simulink library "LM_LIB"  (R2019b)
settings: Solver=VariableStepAuto  StartTime=0.0  StopTime=10.0  RelTol=1e-3
undefined symbols (not defined in the file): P_LM_FusBLParFiltP, P_LM_FusParC0Index, P_LM_FusParC1Index, P_LM_FusParC2Index, P_LM_FusParC3Index, P_LM_OTLBufTPMinPntNum, P_LM_OTLBufTPSPosMinDis, P_LM_OTLRearMaxDis, P_LM_OTLTPNum
libraries: simulink x84, $bdroot x3
(part 1 of 5)
settings Model: Creator=GW00166374  LastModifiedBy=GW00166374

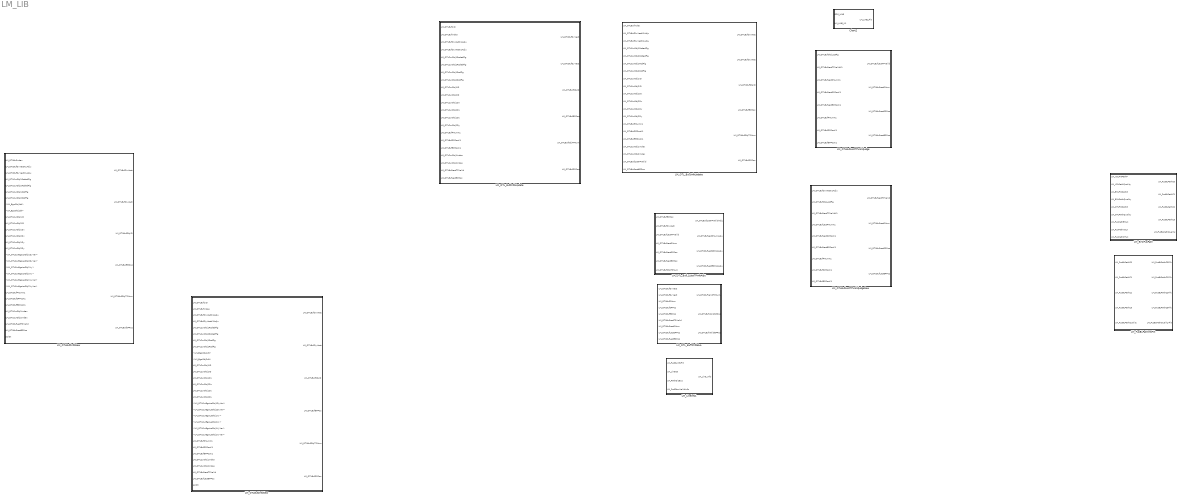
== system LM_LIB ==
  Chart2 : Stateflow chart  TreatAsAtomicUnit=on
  LM_EVOFusPath : Subsystem
  LM_FusBLPathInfoFilt : Subsystem
  LM_LineInfo1 : Subsystem
  LM_OTLBuf1InfoNew : Subsystem
  LM_OTLBuf2InfoNew : Subsystem
  LM_OTLBufLostTPValidJudge : Subsystem
  LM_OTLBufLostTPValidJudgeNew : Subsystem
  LM_OTL_Buf1InfoUpdate : Subsystem
  LM_OTL_Buf2InfoUpdate : Subsystem
  LM_OTL_BufL1LastTPInfoAdju : Subsystem
  LM_OTL_BufTPInfoEva : Subsystem

== system LM_LIB/LM_EVOFusPath ==
  LM_VSLFntPathP : Inport
  LM_VSLPathQuality : Inport  Port=2
  LM_EMLFntPathP : Inport  Port=3
  LM_EMLPathQuality : Inport  Port=4
  LM_OTLFntPathP : Inport  Port=5
  LM_OTLPathQuality : Inport  Port=6
  LM_FusPathEMLK : Inport  Port=7
  LM_FusPathVSLK : Inport  Port=8
  LM_FusPathOTLK : Inport  Port=9
  LM_FusBLPathC0Calc : Subsystem
  LM_FusBLPathC1Calc : Subsystem
  LM_FusBLPathC2Calc : Subsystem
  LM_FusBLPathC3Calc : Subsystem
  LM_FusBLPathQualityCalc : Stateflow chart  BlockKeywords=__PRM__SERIALIZED__DATA__:Stateflow Chart,Stateflow Diagram  TreatAsAtomicUnit=on
  LM_FusBLPathC0 : Outport
  LM_FusBLPathC1 : Outport  Port=2
  LM_FusBLPathC2 : Outport  Port=3
  LM_FusBLPathC3 : Outport  Port=4
  LM_FusBLPathQuality : Outport  Port=5
  wires:
  LM_FusBLPathQualityCalc/1(LM_FusBLPathQuality) -> LM_FusBLPathQuality/1, [LM_FusBLPathQuality]
  LM_FusBLPathC3Calc/1(LM_FusBLPathC3) -> LM_FusBLPathC3/1
  LM_FusBLPathC2Calc/1(LM_FusBLPathC2) -> LM_FusBLPathC2/1
  LM_FusBLPathC1Calc/1(LM_FusBLPathC1) -> LM_FusBLPathC1/1
  LM_FusBLPathC0Calc/1(LM_FusBLPathC0) -> LM_FusBLPathC0/1
  LM_OTLPathQuality/1 -> LM_FusBLPathQualityCalc/3(LM_OTLPathQuality)
  LM_EMLPathQuality/1 -> LM_FusBLPathQualityCalc/1(LM_EMLPathQuality)
  LM_VSLPathQuality/1 -> LM_FusBLPathQualityCalc/2(LM_VSLPathQuality)
  LM_FusPathOTLK/1 -> LM_FusBLPathC3Calc/7(LM_FusPathOTLK), LM_FusBLPathC2Calc/7(LM_FusPathOTLK), LM_FusBLPathC1Calc/7(LM_FusPathOTLK), LM_FusBLPathC0Calc/7(LM_FusPathOTLK), LM_FusBLPathQualityCalc/6(LM_FusPathOTLK)
  LM_FusPathVSLK/1 -> LM_FusBLPathC3Calc/6(LM_FusPathVSLK), LM_FusBLPathC2Calc/6(LM_FusPathVSLK), LM_FusBLPathC1Calc/6(LM_FusPathVSLK), LM_FusBLPathC0Calc/6(LM_FusPathVSLK), LM_FusBLPathQualityCalc/5(LM_FusPathVSLK)
  LM_FusPathEMLK/1 -> LM_FusBLPathC3Calc/5(LM_FusPathEMLK), LM_FusBLPathC2Calc/5(LM_FusPathEMLK), LM_FusBLPathC1Calc/5(LM_FusPathEMLK), LM_FusBLPathC0Calc/5(LM_FusPathEMLK), LM_FusBLPathQualityCalc/4(LM_FusPathEMLK)
  LM_OTLFntPathP/1 -> LM_FusBLPathC1Calc/4(LM_OTLPathP), LM_FusBLPathC2Calc/4(LM_OTLPathP), LM_FusBLPathC3Calc/4(LM_OTLPathP), LM_FusBLPathC0Calc/4(LM_OTLPathP)
  LM_EMLFntPathP/1 -> LM_FusBLPathC1Calc/3(LM_EMLPathP), LM_FusBLPathC2Calc/3(LM_EMLPathP), LM_FusBLPathC3Calc/3(LM_EMLPathP), LM_FusBLPathC0Calc/3(LM_EMLPathP)
  LM_VSLFntPathP/1 -> LM_FusBLPathC0Calc/2(LM_VSLPathP), LM_FusBLPathC1Calc/2(LM_VSLPathP), LM_FusBLPathC2Calc/2(LM_VSLPathP), LM_FusBLPathC3Calc/2(LM_VSLPathP)
  [LM_FusBLPathQuality] -> LM_FusBLPathC0Calc/1(LM_FusBLPathQuality), LM_FusBLPathC1Calc/1(LM_FusBLPathQuality), LM_FusBLPathC2Calc/1(LM_FusBLPathQuality), LM_FusBLPathC3Calc/1(LM_FusBLPathQuality)

== system LM_LIB/LM_FusBLPathInfoFilt ==
  LM_FusBLPathC0 : Inport
  LM_FusBLPathC1 : Inport  Port=2
  LM_FusBLPathC2 : Inport  Port=3
  LM_FusBLPathC3 : Inport  Port=4
  LM_FusBLPathQuality : Inport  Port=5
  LM_FusBLPathQuliatyFilt : Subsystem
  LM_Fus_BLFntPathC0Filt : Subsystem
  LM_Fus_BLPath3C3Filt : Subsystem
  LM_Fus_BLPathC1Filt : Subsystem
  LM_Fus_BLPathC2Filt : Subsystem
  Unit Delay{,1..4} (5 alike) : UnitDelay  SampleTime=-1  HasFrameUpgradeWarning=on
  LM_FusBLPathC0Filt : Outport
  LM_FusBLPathC1Filt : Outport  Port=2
  LM_FusBLPathC2Filt : Outport  Port=3
  LM_FusBLPathC3Filt : Outport  Port=4
  LM_FusBLPathQualityFilt : Outport  Port=5
  wires:
  LM_FusBLPathQuliatyFilt/1(LM_FusBLPathQualityFilt) -> Unit Delay4/1, LM_FusBLPathQualityFilt/1
  LM_Fus_BLPath3C3Filt/1(LM_FusBLPathC3Filt) -> Unit Delay3/1, LM_FusBLPathC3Filt/1
  Unit Delay3/1 -> LM_Fus_BLPath3C3Filt/4(LM_FusBLPathC3K1)
  LM_FusBLPathC3/1 -> LM_Fus_BLPath3C3Filt/3(LM_FusBLPathC3BefFilt)
  LM_Fus_BLPathC2Filt/1(LM_FusBLPathC2Filt) -> Unit Delay2/1, LM_FusBLPathC2Filt/1
  Unit Delay2/1 -> LM_Fus_BLPathC2Filt/4(LM_FusBLPathC2K1)
  LM_FusBLPathC2/1 -> LM_Fus_BLPathC2Filt/3(LM_FusBLPathC2BefFilt)
  Unit Delay1/1 -> LM_Fus_BLPathC1Filt/4(LM_FusBLPathC1K1)
  Unit Delay4/1 -> LM_FusBLPathQuliatyFilt/2(LM_FusBLPathQualityK1), LM_Fus_BLFntPathC0Filt/3(LM_FusBLPathQualityK1), LM_Fus_BLPathC1Filt/1(LM_FusBLPathQualityK1), LM_Fus_BLPathC2Filt/1(LM_FusBLPathQualityK1), LM_Fus_BLPath3C3Filt/1(LM_FusBLPathQualityK1)
  LM_FusBLPathC1/1 -> LM_Fus_BLPathC1Filt/3(LM_FusBLPathC1BefFilt)
  Unit Delay/1 -> LM_Fus_BLFntPathC0Filt/4(LM_FusBLPathC0K1)
  LM_FusBLPathQuality/1 -> LM_Fus_BLFntPathC0Filt/2(LM_FusBLPathQuality), LM_Fus_BLPathC1Filt/2(LM_FusBLPathQuality), LM_Fus_BLPathC2Filt/2(LM_FusBLPathQuality), LM_Fus_BLPath3C3Filt/2(LM_FusBLPathQuality), LM_FusBLPathQuliatyFilt/1(LM_FusBLPathQuality)
  LM_FusBLPathC0/1 -> LM_Fus_BLFntPathC0Filt/1(LM_FusBLPathC0)
  LM_Fus_BLFntPathC0Filt/1(LM_FusBLPathC0Filt) -> LM_FusBLPathC0Filt/1, Unit Delay/1
  LM_Fus_BLPathC1Filt/1(LM_FusBLPathC1Filt) -> LM_FusBLPathC1Filt/1, Unit Delay1/1

== system LM_LIB/LM_LineInfo1 ==
  LM_FusBLInfoFilt : Inport
  LM_LineC0 : Inport  Port=2
  LM_PathDisBus : Inport  Port=3
  LM_FusfCamValidInfo : Inport  Port=4
  Bus Creator1 : BusCreator  Inputs=8  OutDataTypeStr=Bus: LM_LINE_BUS  NonVirtualBus=on
  LM_Line_Fnt : Subsystem
  LM_Line_Rear : Subsystem
  LM_Line_Info : Outport
  wires:
  LM_Line_Fnt/1(LM_Line04) -> Bus Creator1/4
  LM_Line_Fnt/5(LM_LL_Line08) -> Bus Creator1/8
  LM_LineC0/1 -> LM_Line_Fnt/1(LM_LineC0), LM_Line_Rear/3(LM_LineC0)
  LM_Line_Fnt/2(LM_Line05) -> Bus Creator1/5
  LM_Line_Rear/3(LM_Line03) -> Bus Creator1/3
  LM_Line_Rear/1(LM_Line01) -> Bus Creator1/1
  LM_Line_Fnt/3(LM_LL_Line06) -> Bus Creator1/6
  LM_Line_Fnt/4(LM_LL_Line07) -> Bus Creator1/7
  Bus Creator1/1 -> LM_Line_Info/1  "LM_Line_Info"
  LM_Line_Rear/2(LM_Line02) -> Bus Creator1/2
  LM_FusBLInfoFilt/1 -> LM_Line_Fnt/3(LM_FusBLInfoFilt), LM_Line_Rear/1(LM_FusBLInfoFilt)
  LM_PathDisBus/1 -> LM_Line_Fnt/2(LM_PathDisBus), LM_Line_Rear/2(LM_PathDisBus)
  LM_FusfCamValidInfo/1 -> LM_Line_Fnt/4(LM_FusfCamValidInfo)

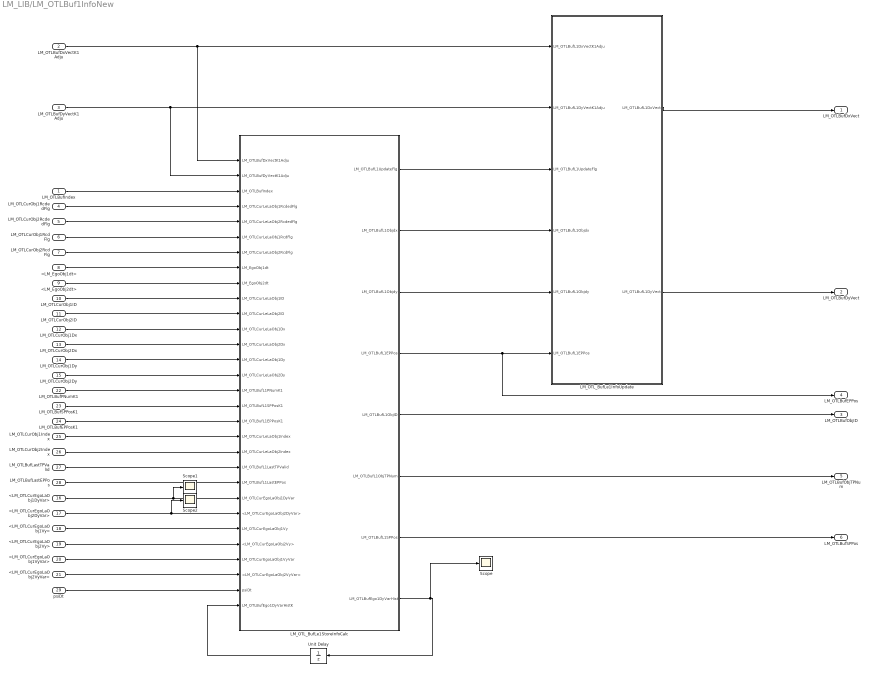
== system LM_LIB/LM_OTLBuf1InfoNew ==
  LM_OTLBufIndex : Inport
  LM_OTLBufDxVectK1Adju : Inport  Port=2
  LM_OTLBufDyVectK1Adju : Inport  Port=3
  LM_OTLCurObj1RcdedFlg : Inport  Port=4
  LM_OTLCurObj2RcdedFlg : Inport  Port=5
  LM_OTLCurObj1RcdFlg : Inport  Port=6
  LM_OTLCurObj2RcdFlg : Inport  Port=7
  <LM_EgoObj1dt> : Inport  Port=8
  <LM_EgoObj2dt> : Inport  Port=9
  LM_OTLCurObj1ID : Inport  Port=10
  LM_OTLCurObj2ID : Inport  Port=11
  LM_OTLCurObj1Dx : Inport  Port=12
  LM_OTLCurObj2Dx : Inport  Port=13
  LM_OTLCurObj1Dy : Inport  Port=14
  LM_OTLCurObj2Dy : Inport  Port=15
  <LM_OTLCurEgoLaObj1DyVar> : Inport  Port=16
  <LM_OTLCurEgoLaObj2DyVar> : Inport  Port=17
  <LM_OTLCurEgoLaObj1Vy> : Inport  Port=18
  <LM_OTLCurEgoLaObj2Vy> : Inport  Port=19
  <LM_OTLCurEgoLaObj1VyVar> : Inport  Port=20
  <LM_OTLCurEgoLaObj2VyVar> : Inport  Port=21
  LM_OTLBufPNumK1 : Inport  Port=22
  LM_OTLBufSPPosK1 : Inport  Port=23
  LM_OTLBufEPPosK1 : Inport  Port=24
  LM_OTLCurObj1Index : Inport  Port=25
  LM_OTLCurObj2Index : Inport  Port=26
  LM_OTLBufLastTPValid : Inport  Port=27
  LM_OTLBufLastEPPos : Inport  Port=28
  psiDt : Inport  Port=29
  LM_OTL_BufLe1InfoUpdate : Subsystem
  LM_OTL_BufLe1StoreInfoCalc : Subsystem
  Scope : Scope
  Scope1 : Scope
  Scope2 : Scope
  Unit Delay : UnitDelay  SampleTime=-1  HasFrameUpgradeWarning=on
  LM_OTLBufDxVect : Outport
  LM_OTLBufDyVect : Outport  Port=2
  LM_OTLBufObjID : Outport  Port=3  OutDataTypeStr=uint8  PortDimensions=1
  LM_OTLBufEPPos : Outport  Port=4  OutDataTypeStr=uint8  PortDimensions=1
  LM_OTLBufObjTPNum : Outport  Port=5  OutDataTypeStr=uint8  PortDimensions=1
  LM_OTLBufSPPos : Outport  Port=6  OutDataTypeStr=uint8  PortDimensions=1
  wires:
  LM_OTL_BufLe1InfoUpdate/2(LM_OTLBufL1DyVect) -> LM_OTLBufDyVect/1
  LM_OTLBufEPPosK1/1 -> LM_OTL_BufLe1StoreInfoCalc/18(LM_OTLBufL1EPPosK1)
  LM_OTLBufIndex/1 -> LM_OTL_BufLe1StoreInfoCalc/3(LM_OTLBufIndex)
  LM_OTLCurObj1Dx/1 -> LM_OTL_BufLe1StoreInfoCalc/12(LM_OTLCurLeLaObj1Dx)
  LM_OTL_BufLe1StoreInfoCalc/7(LM_OTLBufL1SPPos) -> LM_OTLBufSPPos/1
  Unit Delay/1 -> LM_OTL_BufLe1StoreInfoCalc/30(LM_OTLBufEgo1DyVarHistK)
  LM_OTL_BufLe1StoreInfoCalc/5(LM_OTLBufL1ObjID) -> LM_OTLBufObjID/1
  <LM_OTLCurEgoLaObj1DyVar>/1 -> Scope1/1, LM_OTL_BufLe1StoreInfoCalc/23(LM_OTLCurEgoLaObj1DyVar)
  psiDt/1 -> LM_OTL_BufLe1StoreInfoCalc/29(psiDt)
  LM_OTLCurObj2Dx/1 -> LM_OTL_BufLe1StoreInfoCalc/13(LM_OTLCurLeLaObj2Dx)
  LM_OTL_BufLe1StoreInfoCalc/4(LM_OTLBufL1EPPos) -> LM_OTLBufEPPos/1, LM_OTL_BufLe1InfoUpdate/6(LM_OTLBufL1EPPos)
  LM_OTLCurObj2RcdFlg/1 -> LM_OTL_BufLe1StoreInfoCalc/7(LM_OTLCurLeLaObj2RcdFlg)
  LM_OTLBufLastEPPos/1 -> LM_OTL_BufLe1StoreInfoCalc/22(LM_OTLBufL1LastEPPos)
  LM_OTL_BufLe1StoreInfoCalc/1(LM_OTLBufL1UpdateFlg) -> LM_OTL_BufLe1InfoUpdate/3(LM_OTLBufL1UpdateFlg)
  <LM_OTLCurEgoLaObj2DyVar>/1 -> Scope2/1, LM_OTL_BufLe1StoreInfoCalc/24(<LM_OTLCurEgoLaObj2DyVar>)
  LM_OTL_BufLe1StoreInfoCalc/3(LM_OTLBufL1Objdy) -> LM_OTL_BufLe1InfoUpdate/5(LM_OTLBufL1Objdy)
  LM_OTL_BufLe1StoreInfoCalc/6(LM_OTLBufL1ObjTPNum) -> LM_OTLBufObjTPNum/1
  LM_OTLBufSPPosK1/1 -> LM_OTL_BufLe1StoreInfoCalc/17(LM_OTLBufL1SPPosK1)
  LM_OTLCurObj1RcdedFlg/1 -> LM_OTL_BufLe1StoreInfoCalc/4(LM_OTLCurLeLaObj1RcdedFlg)
  LM_OTLCurObj1ID/1 -> LM_OTL_BufLe1StoreInfoCalc/10(LM_OTLCurLeLaObj1ID)
  LM_OTLCurObj2RcdedFlg/1 -> LM_OTL_BufLe1StoreInfoCalc/5(LM_OTLCurLeLaObj2RcdedFlg)
  LM_OTL_BufLe1InfoUpdate/1(LM_OTLBufL1DxVect) -> LM_OTLBufDxVect/1
  LM_OTLBufDyVectK1Adju/1 -> LM_OTL_BufLe1StoreInfoCalc/2(LM_OTLBufDyVectK1Adju), LM_OTL_BufLe1InfoUpdate/2(LM_OTLBufL1DyVectK1Adju)
  LM_OTLCurObj2Index/1 -> LM_OTL_BufLe1StoreInfoCalc/20(LM_OTLCurLeLaObj2Index)
  LM_OTLCurObj2Dy/1 -> LM_OTL_BufLe1StoreInfoCalc/15(LM_OTLCurLeLaObj2Dy)
  LM_OTLBufLastTPValid/1 -> LM_OTL_BufLe1StoreInfoCalc/21(LM_OTLBufL1LastTPValid)
  LM_OTLCurObj1Dy/1 -> LM_OTL_BufLe1StoreInfoCalc/14(LM_OTLCurLeLaObj1Dy)
  LM_OTLBufPNumK1/1 -> LM_OTL_BufLe1StoreInfoCalc/16(LM_OTLBufL1PNumK1)
  <LM_EgoObj1dt>/1 -> LM_OTL_BufLe1StoreInfoCalc/8(LM_EgoObj1dt)
  LM_OTL_BufLe1StoreInfoCalc/2(LM_OTLBufL1Objdx) -> LM_OTL_BufLe1InfoUpdate/4(LM_OTLBufL1Objdx)
  <LM_OTLCurEgoLaObj1VyVar>/1 -> LM_OTL_BufLe1StoreInfoCalc/27(LM_OTLCurEgoLaObj1VyVar)
  LM_OTLCurObj2ID/1 -> LM_OTL_BufLe1StoreInfoCalc/11(LM_OTLCurLeLaObj2ID)
  LM_OTLBufDxVectK1Adju/1 -> LM_OTL_BufLe1StoreInfoCalc/1(LM_OTLBufDxVectK1Adju), LM_OTL_BufLe1InfoUpdate/1(LM_OTLBufL1DxVectK1Adju)
  <LM_OTLCurEgoLaObj2Vy>/1 -> LM_OTL_BufLe1StoreInfoCalc/26(<LM_OTLCurEgoLaObj2Vy>)
  LM_OTLCurObj1Index/1 -> LM_OTL_BufLe1StoreInfoCalc/19(LM_OTLCurLeLaObj1Index)
  <LM_OTLCurEgoLaObj2VyVar>/1 -> LM_OTL_BufLe1StoreInfoCalc/28(<LM_OTLCurEgoLaObj2VyVar>)
  <LM_EgoObj2dt>/1 -> LM_OTL_BufLe1StoreInfoCalc/9(LM_EgoObj2dt)
  <LM_OTLCurEgoLaObj1Vy>/1 -> LM_OTL_BufLe1StoreInfoCalc/25(LM_OTLCurEgoLaObj1Vy)
  LM_OTLCurObj1RcdFlg/1 -> LM_OTL_BufLe1StoreInfoCalc/6(LM_OTLCurLeLaObj1RcdFlg)
  LM_OTL_BufLe1StoreInfoCalc/8(LM_OTLBufEgo1DyVarHist) -> Scope/1, Unit Delay/1

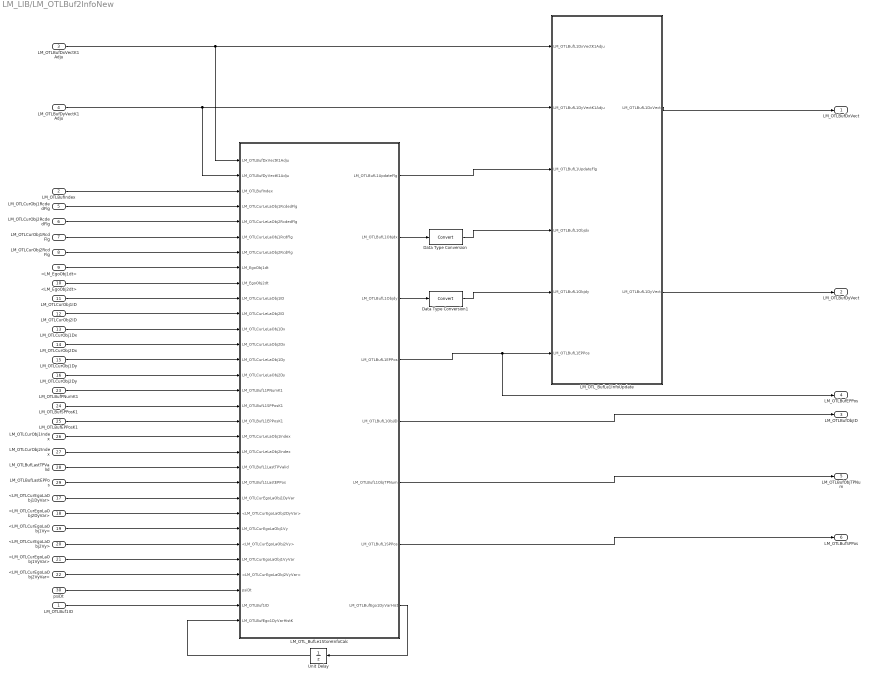
== system LM_LIB/LM_OTLBuf2InfoNew ==
  LM_OTLBuf1ID : Inport
  LM_OTLBufIndex : Inport  Port=2
  LM_OTLBufDxVectK1Adju : Inport  Port=3
  LM_OTLBufDyVectK1Adju : Inport  Port=4
  LM_OTLCurObj1RcdedFlg : Inport  Port=5
  LM_OTLCurObj2RcdedFlg : Inport  Port=6
  LM_OTLCurObj1RcdFlg : Inport  Port=7
  LM_OTLCurObj2RcdFlg : Inport  Port=8
  <LM_EgoObj1dt> : Inport  Port=9
  <LM_EgoObj2dt> : Inport  Port=10
  LM_OTLCurObj1ID : Inport  Port=11
  LM_OTLCurObj2ID : Inport  Port=12
  LM_OTLCurObj1Dx : Inport  Port=13
  LM_OTLCurObj2Dx : Inport  Port=14
  LM_OTLCurObj1Dy : Inport  Port=15
  LM_OTLCurObj2Dy : Inport  Port=16
  <LM_OTLCurEgoLaObj1DyVar> : Inport  Port=17
  <LM_OTLCurEgoLaObj2DyVar> : Inport  Port=18
  <LM_OTLCurEgoLaObj1Vy> : Inport  Port=19
  <LM_OTLCurEgoLaObj2Vy> : Inport  Port=20
  <LM_OTLCurEgoLaObj1VyVar> : Inport  Port=21
  <LM_OTLCurEgoLaObj2VyVar> : Inport  Port=22
  LM_OTLBufPNumK1 : Inport  Port=23
  LM_OTLBufSPPosK1 : Inport  Port=24
  LM_OTLBufEPPosK1 : Inport  Port=25
  LM_OTLCurObj1Index : Inport  Port=26
  LM_OTLCurObj2Index : Inport  Port=27
  LM_OTLBufLastTPValid : Inport  Port=28
  LM_OTLBufLastEPPos : Inport  Port=29
  psiDt : Inport  Port=30
  Data Type Conversion : DataTypeConversion
  Data Type Conversion1 : DataTypeConversion
  LM_OTL_BufLe1InfoUpdate : Subsystem
  LM_OTL_BufLe1StoreInfoCalc : Subsystem
  Unit Delay : UnitDelay  SampleTime=-1  HasFrameUpgradeWarning=on
  LM_OTLBufDxVect : Outport
  LM_OTLBufDyVect : Outport  Port=2
  LM_OTLBufObjID : Outport  Port=3  OutDataTypeStr=uint8  PortDimensions=1
  LM_OTLBufEPPos : Outport  Port=4  OutDataTypeStr=uint8  PortDimensions=1
  LM_OTLBufObjTPNum : Outport  Port=5  OutDataTypeStr=uint8  PortDimensions=1
  LM_OTLBufSPPos : Outport  Port=6  OutDataTypeStr=uint8  PortDimensions=1
  wires:
  LM_OTL_BufLe1InfoUpdate/2(LM_OTLBufL1DyVect) -> LM_OTLBufDyVect/1
  LM_OTLBufEPPosK1/1 -> LM_OTL_BufLe1StoreInfoCalc/18(LM_OTLBufL1EPPosK1)
  LM_OTLBufIndex/1 -> LM_OTL_BufLe1StoreInfoCalc/3(LM_OTLBufIndex)
  LM_OTLCurObj1Dx/1 -> LM_OTL_BufLe1StoreInfoCalc/12(LM_OTLCurLeLaObj1Dx)
  LM_OTL_BufLe1StoreInfoCalc/7(LM_OTLBufL1SPPos) -> LM_OTLBufSPPos/1
  Unit Delay/1 -> LM_OTL_BufLe1StoreInfoCalc/31(LM_OTLBufEgo1DyVarHistK)
  LM_OTL_BufLe1StoreInfoCalc/5(LM_OTLBufL1ObjID) -> LM_OTLBufObjID/1
  <LM_OTLCurEgoLaObj1DyVar>/1 -> LM_OTL_BufLe1StoreInfoCalc/23(LM_OTLCurEgoLaObj1DyVar)
  psiDt/1 -> LM_OTL_BufLe1StoreInfoCalc/29(psiDt)
  LM_OTLCurObj2Dx/1 -> LM_OTL_BufLe1StoreInfoCalc/13(LM_OTLCurLeLaObj2Dx)
  LM_OTL_BufLe1StoreInfoCalc/4(LM_OTLBufL1EPPos) -> LM_OTLBufEPPos/1, LM_OTL_BufLe1InfoUpdate/6(LM_OTLBufL1EPPos)
  LM_OTLCurObj2RcdFlg/1 -> LM_OTL_BufLe1StoreInfoCalc/7(LM_OTLCurLeLaObj2RcdFlg)
  LM_OTLBufLastEPPos/1 -> LM_OTL_BufLe1StoreInfoCalc/22(LM_OTLBufL1LastEPPos)
  LM_OTL_BufLe1StoreInfoCalc/1(LM_OTLBufL1UpdateFlg) -> LM_OTL_BufLe1InfoUpdate/3(LM_OTLBufL1UpdateFlg)
  <LM_OTLCurEgoLaObj2DyVar>/1 -> LM_OTL_BufLe1StoreInfoCalc/24(<LM_OTLCurEgoLaObj2DyVar>)
  LM_OTL_BufLe1StoreInfoCalc/3(LM_OTLBufL1Objdy) -> Data Type Conversion1/1
  LM_OTL_BufLe1StoreInfoCalc/6(LM_OTLBufL1ObjTPNum) -> LM_OTLBufObjTPNum/1
  LM_OTLBufSPPosK1/1 -> LM_OTL_BufLe1StoreInfoCalc/17(LM_OTLBufL1SPPosK1)
  LM_OTLCurObj1RcdedFlg/1 -> LM_OTL_BufLe1StoreInfoCalc/4(LM_OTLCurLeLaObj1RcdedFlg)
  LM_OTLCurObj1ID/1 -> LM_OTL_BufLe1StoreInfoCalc/10(LM_OTLCurLeLaObj1ID)
  LM_OTLCurObj2RcdedFlg/1 -> LM_OTL_BufLe1StoreInfoCalc/5(LM_OTLCurLeLaObj2RcdedFlg)
  LM_OTL_BufLe1InfoUpdate/1(LM_OTLBufL1DxVect) -> LM_OTLBufDxVect/1
  LM_OTLBufDyVectK1Adju/1 -> LM_OTL_BufLe1StoreInfoCalc/2(LM_OTLBufDyVectK1Adju), LM_OTL_BufLe1InfoUpdate/2(LM_OTLBufL1DyVectK1Adju)
  LM_OTLCurObj2Index/1 -> LM_OTL_BufLe1StoreInfoCalc/20(LM_OTLCurLeLaObj2Index)
  LM_OTLCurObj2Dy/1 -> LM_OTL_BufLe1StoreInfoCalc/15(LM_OTLCurLeLaObj2Dy)
  LM_OTLBufLastTPValid/1 -> LM_OTL_BufLe1StoreInfoCalc/21(LM_OTLBufL1LastTPValid)
  LM_OTLCurObj1Dy/1 -> LM_OTL_BufLe1StoreInfoCalc/14(LM_OTLCurLeLaObj1Dy)
  LM_OTLBufPNumK1/1 -> LM_OTL_BufLe1StoreInfoCalc/16(LM_OTLBufL1PNumK1)
  <LM_EgoObj1dt>/1 -> LM_OTL_BufLe1StoreInfoCalc/8(LM_EgoObj1dt)
  LM_OTL_BufLe1StoreInfoCalc/2(LM_OTLBufL1Objdx) -> Data Type Conversion/1
  <LM_OTLCurEgoLaObj1VyVar>/1 -> LM_OTL_BufLe1StoreInfoCalc/27(LM_OTLCurEgoLaObj1VyVar)
  LM_OTLCurObj2ID/1 -> LM_OTL_BufLe1StoreInfoCalc/11(LM_OTLCurLeLaObj2ID)
  LM_OTLBufDxVectK1Adju/1 -> LM_OTL_BufLe1StoreInfoCalc/1(LM_OTLBufDxVectK1Adju), LM_OTL_BufLe1InfoUpdate/1(LM_OTLBufL1DxVectK1Adju)
  <LM_OTLCurEgoLaObj2Vy>/1 -> LM_OTL_BufLe1StoreInfoCalc/26(<LM_OTLCurEgoLaObj2Vy>)
  LM_OTLCurObj1Index/1 -> LM_OTL_BufLe1StoreInfoCalc/19(LM_OTLCurLeLaObj1Index)
  <LM_OTLCurEgoLaObj2VyVar>/1 -> LM_OTL_BufLe1StoreInfoCalc/28(<LM_OTLCurEgoLaObj2VyVar>)
  <LM_EgoObj2dt>/1 -> LM_OTL_BufLe1StoreInfoCalc/9(LM_EgoObj2dt)
  <LM_OTLCurEgoLaObj1Vy>/1 -> LM_OTL_BufLe1StoreInfoCalc/25(LM_OTLCurEgoLaObj1Vy)
  LM_OTLCurObj1RcdFlg/1 -> LM_OTL_BufLe1StoreInfoCalc/6(LM_OTLCurLeLaObj1RcdFlg)
  LM_OTL_BufLe1StoreInfoCalc/8(LM_OTLBufEgo1DyVarHist) -> Unit Delay/1
  LM_OTLBuf1ID/1 -> LM_OTL_BufLe1StoreInfoCalc/30(LM_OTLBuf1ID)
  Data Type Conversion/1 -> LM_OTL_BufLe1InfoUpdate/4(LM_OTLBufL1Objdx)
  Data Type Conversion1/1 -> LM_OTL_BufLe1InfoUpdate/5(LM_OTLBufL1Objdy)

== system LM_LIB/LM_OTLBufLostTPValidJudge ==
  LM_OTLBufObjLostFlg : Inport
  LM_OTLBufLastTPValidK1 : Inport  Port=2
  LM_OTLBufLastPNumK1 : Inport  Port=3
  LM_OTLBufLastSPPosK1 : Inport  Port=4
  LM_OTLBufLastEPPosK1 : Inport  Port=5
  LM_OTLBufPNumK1 : Inport  Port=6
  LM_OTLBufSPPosK1 : Inport  Port=7
  LM_OTLBufEPPosK1 : Inport  Port=8
  Constant : Constant  Value=15
  Constant1 : Constant  OutDataTypeStr=uint8
  Constant{2..5} (4 alike) : Constant  Value=0  OutDataTypeStr=uint8
  DocBlock : simulink/Model-Wide Utilities/DocBlock  DocumentType=Text
      content=|
      | 1. Function Description
      |    在buffer中存储的目标丢失时，判断其buffer中存的历史轨迹点是否有效
      | 2. Algorithm Description
      |    当buffer中的存储目标丢失时
      |    1)如果当前上一存储目标轨迹无效
      |    判断存储的历史轨迹在本车前方的有效长度是否大于10m，如果大于则该buffer中上一目标历史轨迹点有效，否则无效
      |    2)如果当前上一存储目标轨迹有效
      |    判断当前丢失的目标的历史轨迹在本车前方的有效长度是否大于10m，如果大于则该buffer中上一目标历史轨迹点有效，否则，判断上上一目标的历史轨迹在本车前方的有效长度是否大于10m，如果大于则该buffer上一目标历史轨迹点有效，其起始位置及轨迹点个数均为上上个存储目标的信息，否则该buffer中的上一目标历史轨迹无效
      | 3. Change Record
  Relational Operator : RelationalOperator  OutDataTypeStr=boolean  RndMeth=Simplest
  Switch{,1..7} (8 alike) : Switch  Criteria=u2 ~= 0
  LM_OTLBufLastTPValid : Outport
  LM_OTLBufLastPNum : Outport  Port=2
  LM_OTLBufLastSPPos : Outport  Port=3
  LM_OTLBufLastEPPos : Outport  Port=4
  wires:
  LM_OTLBufLastEPPosK1/1 -> Switch6/3
  Constant5/1 -> Switch7/3
  LM_OTLBufEPPosK1/1 -> Switch7/1
  Switch7/1 -> Switch6/1
  Switch6/1 -> LM_OTLBufLastEPPos/1
  LM_OTLBufLastSPPosK1/1 -> Switch4/3
  Constant4/1 -> Switch5/3
  LM_OTLBufSPPosK1/1 -> Switch5/1
  Switch5/1 -> Switch4/1
  Switch4/1 -> LM_OTLBufLastSPPos/1
  LM_OTLBufLastPNumK1/1 -> Switch3/3
  Switch3/1 -> LM_OTLBufLastPNum/1
  Switch2/1 -> Switch3/1
  Constant3/1 -> Switch2/3
  Switch/1 -> LM_OTLBufLastTPValid/1
  LM_OTLBufLastTPValidK1/1 -> Switch/3
  Switch1/1 -> Switch/1
  Constant2/1 -> Switch1/3
  Constant1/1 -> Switch1/1
  Relational Operator/1 -> Switch1/2, Switch2/2, Switch7/2, Switch5/2
  Constant/1 -> Relational Operator/2
  LM_OTLBufPNumK1/1 -> Relational Operator/1, Switch2/1
  LM_OTLBufObjLostFlg/1 -> Switch/2, Switch4/2, Switch6/2, Switch3/2

== system LM_LIB/LM_OTLBufLostTPValidJudgeNew ==
  LM_OTLBufDxVectK1Adju : Inport
  LM_OTLBufObjLostFlg : Inport  Port=2
  LM_OTLBufLastTPValidK1 : Inport  Port=3
  LM_OTLBufLastPNumK1 : Inport  Port=4
  LM_OTLBufLastSPPosK1 : Inport  Port=5
  LM_OTLBufLastEPPosK1 : Inport  Port=6
  LM_OTLBufPNumK1 : Inport  Port=7
  LM_OTLBufSPPosK1 : Inport  Port=8
  LM_OTLBufEPPosK1 : Inport  Port=9
  DocBlock : simulink/Model-Wide Utilities/DocBlock  DocumentType=Text
      content=|
      | Type your documentation here
  If : If  IfExpression=u1 ~= 0
  If Action Subsystem : Subsystem  TreatAsAtomicUnit=on
  If Action Subsystem1 : Subsystem  TreatAsAtomicUnit=on
  Merge{,1..3} (4 alike) : Merge
  LM_OTLBufLastTPValid : Outport
  LM_OTLBufLastPNum : Outport  Port=2
  LM_OTLBufLastSPPos : Outport  Port=3
  LM_OTLBufLastEPPos : Outport  Port=4
  wires:
  LM_OTLBufObjLostFlg/1 -> If/1
  If/1 -> If Action Subsystem/Action
  If/2 -> If Action Subsystem1/Action
  LM_OTLBufDxVectK1Adju/1 -> If Action Subsystem/1(LM_OTLBufL1DxVectK1Adju)
  LM_OTLBufPNumK1/1 -> If Action Subsystem/2(LM_OTLBufPNumK1)
  LM_OTLBufSPPosK1/1 -> If Action Subsystem/3(LM_OTLBufSPPosK1)
  LM_OTLBufEPPosK1/1 -> If Action Subsystem/4(LM_OTLBufEPPosK1)
  LM_OTLBufLastTPValidK1/1 -> If Action Subsystem1/1(LM_OTLBufLastTPValidK1), If Action Subsystem/5(LM_OTLBufLastTPValidK1)
  LM_OTLBufLastPNumK1/1 -> If Action Subsystem1/2(LM_OTLBufLastPNumK1), If Action Subsystem/6(LM_OTLBufLastPNumK1)
  LM_OTLBufLastSPPosK1/1 -> If Action Subsystem1/3(LM_OTLBufLastSPPosK1), If Action Subsystem/7(LM_OTLBufLastSPPosK1)
  LM_OTLBufLastEPPosK1/1 -> If Action Subsystem1/4(LM_OTLBufLastEPPosK1), If Action Subsystem/8(LM_OTLBufLastEPPosK1)
  Merge2/1 -> LM_OTLBufLastSPPos/1  "LM_OTLBufLastSPPos"
  Merge/1 -> LM_OTLBufLastTPValid/1  "LM_OTLBufLastTPValid"
  Merge1/1 -> LM_OTLBufLastPNum/1  "LM_OTLBufLastPNum"
  Merge3/1 -> LM_OTLBufLastEPPos/1  "LM_OTLBufLastEPPos"
  If Action Subsystem/1(LM_OTLBufLastTPValid) -> Merge/1
  If Action Subsystem/2(LM_OTLBufLastPNum) -> Merge1/1
  If Action Subsystem/3(LM_OTLBufLastSPPos) -> Merge2/1
  If Action Subsystem/4(LM_OTLBufLastEPPos) -> Merge3/1
  If Action Subsystem1/1(LM_OTLBufLastTPValid) -> Merge/2
  If Action Subsystem1/2(LM_OTLBufLastPNum) -> Merge1/2
  If Action Subsystem1/3(LM_OTLBufLastSPPos) -> Merge2/2
  If Action Subsystem1/4(LM_OTLBufLastEPPos) -> Merge3/2

== system LM_LIB/LM_OTL_Buf1InfoUpdate ==
  LM_OTLBufIndex : Inport
  LM_OTLBufDxVectK1Adju : Inport  Port=2
  LM_OTLBufDyVectK1Adju : Inport  Port=3
  LM_OTLCurObj1RcdedFlg : Inport  Port=4
  LM_OTLCurObj2RcdedFlg : Inport  Port=5
  LM_OTLCurObj1RcdFlg : Inport  Port=6
  LM_OTLCurObj2RcdFlg : Inport  Port=7
  LM_OTLCurObj1ID : Inport  Port=8
  LM_OTLCurObj2ID : Inport  Port=9
  LM_OTLCurObj1Dx : Inport  Port=10
  LM_OTLCurObj2Dx : Inport  Port=11
  LM_OTLCurObj1Dy : Inport  Port=12
  LM_OTLCurObj2Dy : Inport  Port=13
  LM_OTLBufPNumK1 : Inport  Port=14
  LM_OTLBufSPPosK1 : Inport  Port=15
  LM_OTLBufEPPosK1 : Inport  Port=16
  LM_OTLCurObj1Index : Inport  Port=17
  LM_OTLCurObj2Index : Inport  Port=18
  LM_OTLBufLastTPValid : Inport  Port=19
  LM_OTLBufLastEPPos : Inport  Port=20
  LM_OTL_BufLe1InfoUpdate : Subsystem
  LM_OTL_BufLe1StoreInfoCalc : Subsystem
  LM_OTLBufDxVect : Outport
  LM_OTLBufDyVect : Outport  Port=2
  LM_OTLBufObjID : Outport  Port=3  OutDataTypeStr=uint8  PortDimensions=1
  LM_OTLBufEPPos : Outport  Port=4  OutDataTypeStr=uint8  PortDimensions=1
  LM_OTLBufObjTPNum : Outport  Port=5  OutDataTypeStr=uint8  PortDimensions=1
  LM_OTLBufSPPos : Outport  Port=6  OutDataTypeStr=uint8  PortDimensions=1
  wires:
  LM_OTLBufIndex/1 -> LM_OTL_BufLe1StoreInfoCalc/2(LM_OTLBufIndex)
  LM_OTLBufDxVectK1Adju/1 -> LM_OTL_BufLe1StoreInfoCalc/1(LM_OTLBufDxVectK1Adju), LM_OTL_BufLe1InfoUpdate/1(LM_OTLBufL1DxVectK1Adju)
  LM_OTLCurObj1Dx/1 -> LM_OTL_BufLe1StoreInfoCalc/9(LM_OTLCurLeLaObj1Dx)
  LM_OTL_BufLe1StoreInfoCalc/5(LM_OTLBufL1ObjID) -> LM_OTLBufObjID/1
  LM_OTL_BufLe1StoreInfoCalc/2(LM_OTLBufL1Objdx) -> LM_OTL_BufLe1InfoUpdate/4(LM_OTLBufL1Objdx)
  LM_OTL_BufLe1StoreInfoCalc/7(LM_OTLBufL1SPPos) -> LM_OTLBufSPPos/1
  LM_OTLBufEPPosK1/1 -> LM_OTL_BufLe1StoreInfoCalc/15(LM_OTLBufL1EPPosK1)
  LM_OTL_BufLe1InfoUpdate/1(LM_OTLBufL1DxVect) -> LM_OTLBufDxVect/1
  LM_OTLCurObj1RcdedFlg/1 -> LM_OTL_BufLe1StoreInfoCalc/3(LM_OTLCurLeLaObj1RcdedFlg)
  LM_OTLCurObj1RcdFlg/1 -> LM_OTL_BufLe1StoreInfoCalc/5(LM_OTLCurLeLaObj1RcdFlg)
  LM_OTL_BufLe1InfoUpdate/2(LM_OTLBufL1DyVect) -> LM_OTLBufDyVect/1
  LM_OTLCurObj1Dy/1 -> LM_OTL_BufLe1StoreInfoCalc/11(LM_OTLCurLeLaObj1Dy)
  LM_OTLCurObj2ID/1 -> LM_OTL_BufLe1StoreInfoCalc/8(LM_OTLCurLeLaObj2ID)
  LM_OTL_BufLe1StoreInfoCalc/4(LM_OTLBufL1EPPos) -> LM_OTL_BufLe1InfoUpdate/6(LM_OTLBufL1EPPos), LM_OTLBufEPPos/1
  LM_OTL_BufLe1StoreInfoCalc/6(LM_OTLBufL1ObjTPNum) -> LM_OTLBufObjTPNum/1
  LM_OTLBufSPPosK1/1 -> LM_OTL_BufLe1StoreInfoCalc/14(LM_OTLBufL1SPPosK1)
  LM_OTLBufDyVectK1Adju/1 -> LM_OTL_BufLe1InfoUpdate/2(LM_OTLBufL1DyVectK1Adju)
  LM_OTL_BufLe1StoreInfoCalc/3(LM_OTLBufL1Objdy) -> LM_OTL_BufLe1InfoUpdate/5(LM_OTLBufL1Objdy)
  LM_OTL_BufLe1StoreInfoCalc/1(LM_OTLBufL1UpdateFlg) -> LM_OTL_BufLe1InfoUpdate/3(LM_OTLBufL1UpdateFlg)
  LM_OTLCurObj1ID/1 -> LM_OTL_BufLe1StoreInfoCalc/7(LM_OTLCurLeLaObj1ID)
  LM_OTLCurObj2Dy/1 -> LM_OTL_BufLe1StoreInfoCalc/12(LM_OTLCurLeLaObj2Dy)
  LM_OTLBufPNumK1/1 -> LM_OTL_BufLe1StoreInfoCalc/13(LM_OTLBufL1PNumK1)
  LM_OTLCurObj2Index/1 -> LM_OTL_BufLe1StoreInfoCalc/17(LM_OTLCurLeLaObj2Index)
  LM_OTLCurObj1Index/1 -> LM_OTL_BufLe1StoreInfoCalc/16(LM_OTLCurLeLaObj1Index)
  LM_OTLCurObj2RcdedFlg/1 -> LM_OTL_BufLe1StoreInfoCalc/4(LM_OTLCurLeLaObj2RcdedFlg)
  LM_OTLBufLastTPValid/1 -> LM_OTL_BufLe1StoreInfoCalc/18(LM_OTLBufL1LastTPValid)
  LM_OTLBufLastEPPos/1 -> LM_OTL_BufLe1StoreInfoCalc/19(LM_OTLBufL1LastEPPos)
  LM_OTLCurObj2RcdFlg/1 -> LM_OTL_BufLe1StoreInfoCalc/6(LM_OTLCurLeLaObj2RcdFlg)
  LM_OTLCurObj2Dx/1 -> LM_OTL_BufLe1StoreInfoCalc/10(LM_OTLCurLeLaObj2Dx)

== system LM_LIB/LM_OTL_Buf2InfoUpdate ==
  LM_OTLBuf1ID : Inport
  LM_OTLBufIndex : Inport  Port=2
  LM_OTLBufDxVectK1Adju : Inport  Port=3
  LM_OTLBufDyVectK1Adju : Inport  Port=4
  LM_OTLCurObj1RcdedFlg : Inport  Port=5
  LM_OTLCurObj2RcdedFlg : Inport  Port=6
  LM_OTLCurObj1RcdFlg : Inport  Port=7
  LM_OTLCurObj2RcdFlg : Inport  Port=8
  LM_OTLCurObj1ID : Inport  Port=9
  LM_OTLCurObj2ID : Inport  Port=10
  LM_OTLCurObj1Dx : Inport  Port=11
  LM_OTLCurObj2Dx : Inport  Port=12
  LM_OTLCurObj1Dy : Inport  Port=13
  LM_OTLCurObj2Dy : Inport  Port=14
  LM_OTLBufPNumK1 : Inport  Port=15
  LM_OTLBufSPPosK1 : Inport  Port=16
  LM_OTLBufEPPosK1 : Inport  Port=17
  LM_OTLCurObj1Index : Inport  Port=18
  LM_OTLCurObj2Index : Inport  Port=19
  LM_OTLBufLastTPValid : Inport  Port=20
  LM_OTLBufLastEPPos : Inport  Port=21
  LM_OTL_BufLe1InfoUpdate : Subsystem
  LM_OTL_BufLe1StoreInfoCalc : Subsystem
  LM_OTLBufDxVect : Outport
  LM_OTLBufDyVect : Outport  Port=2
  LM_OTLBufObjID : Outport  Port=3  OutDataTypeStr=uint8  PortDimensions=1
  LM_OTLBufEPPos : Outport  Port=4  OutDataTypeStr=uint8  PortDimensions=1
  LM_OTLBufObjTPNum : Outport  Port=5  OutDataTypeStr=uint8  PortDimensions=1
  LM_OTLBufSPPos : Outport  Port=6  OutDataTypeStr=uint8  PortDimensions=1
  wires:
  LM_OTLBufIndex/1 -> LM_OTL_BufLe1StoreInfoCalc/3(LM_OTLBufIndex)
  LM_OTLBufDxVectK1Adju/1 -> LM_OTL_BufLe1StoreInfoCalc/1(LM_OTLBufDxVectK1Adju), LM_OTL_BufLe1InfoUpdate/1(LM_OTLBufL1DxVectK1Adju)
  LM_OTLCurObj1Dx/1 -> LM_OTL_BufLe1StoreInfoCalc/10(LM_OTLCurLeLaObj1Dx)
  LM_OTL_BufLe1StoreInfoCalc/5(LM_OTLBufL1ObjID) -> LM_OTLBufObjID/1
  LM_OTL_BufLe1StoreInfoCalc/2(LM_OTLBufL1Objdx) -> LM_OTL_BufLe1InfoUpdate/4(LM_OTLBufL1Objdx)
  LM_OTL_BufLe1StoreInfoCalc/7(LM_OTLBufL1SPPos) -> LM_OTLBufSPPos/1
  LM_OTLBufEPPosK1/1 -> LM_OTL_BufLe1StoreInfoCalc/16(LM_OTLBufL1EPPosK1)
  LM_OTL_BufLe1InfoUpdate/1(LM_OTLBufL1DxVect) -> LM_OTLBufDxVect/1
  LM_OTLCurObj1RcdedFlg/1 -> LM_OTL_BufLe1StoreInfoCalc/4(LM_OTLCurLeLaObj1RcdedFlg)
  LM_OTLCurObj1RcdFlg/1 -> LM_OTL_BufLe1StoreInfoCalc/6(LM_OTLCurLeLaObj1RcdFlg)
  LM_OTL_BufLe1InfoUpdate/2(LM_OTLBufL1DyVect) -> LM_OTLBufDyVect/1
  LM_OTLCurObj1Dy/1 -> LM_OTL_BufLe1StoreInfoCalc/12(LM_OTLCurLeLaObj1Dy)
  LM_OTLCurObj2ID/1 -> LM_OTL_BufLe1StoreInfoCalc/9(LM_OTLCurLeLaObj2ID)
  LM_OTL_BufLe1StoreInfoCalc/4(LM_OTLBufL1EPPos) -> LM_OTL_BufLe1InfoUpdate/6(LM_OTLBufL1EPPos), LM_OTLBufEPPos/1
  LM_OTL_BufLe1StoreInfoCalc/6(LM_OTLBufL1ObjTPNum) -> LM_OTLBufObjTPNum/1
  LM_OTLBufSPPosK1/1 -> LM_OTL_BufLe1StoreInfoCalc/15(LM_OTLBufL1SPPosK1)
  LM_OTLBufDyVectK1Adju/1 -> LM_OTL_BufLe1InfoUpdate/2(LM_OTLBufL1DyVectK1Adju)
  LM_OTL_BufLe1StoreInfoCalc/3(LM_OTLBufL1Objdy) -> LM_OTL_BufLe1InfoUpdate/5(LM_OTLBufL1Objdy)
  LM_OTL_BufLe1StoreInfoCalc/1(LM_OTLBufL1UpdateFlg) -> LM_OTL_BufLe1InfoUpdate/3(LM_OTLBufL1UpdateFlg)
  LM_OTLCurObj1ID/1 -> LM_OTL_BufLe1StoreInfoCalc/8(LM_OTLCurLeLaObj1ID)
  LM_OTLCurObj2Dy/1 -> LM_OTL_BufLe1StoreInfoCalc/13(LM_OTLCurLeLaObj2Dy)
  LM_OTLBufPNumK1/1 -> LM_OTL_BufLe1StoreInfoCalc/14(LM_OTLBufL1PNumK1)
  LM_OTLCurObj2Index/1 -> LM_OTL_BufLe1StoreInfoCalc/18(LM_OTLCurLeLaObj2Index)
  LM_OTLCurObj1Index/1 -> LM_OTL_BufLe1StoreInfoCalc/17(LM_OTLCurLeLaObj1Index)
  LM_OTLCurObj2RcdedFlg/1 -> LM_OTL_BufLe1StoreInfoCalc/5(LM_OTLCurLeLaObj2RcdedFlg)
  LM_OTLBufLastTPValid/1 -> LM_OTL_BufLe1StoreInfoCalc/19(LM_OTLBufL1LastTPValid)
  LM_OTLBufLastEPPos/1 -> LM_OTL_BufLe1StoreInfoCalc/20(LM_OTLBufL1LastEPPos)
  LM_OTLCurObj2RcdFlg/1 -> LM_OTL_BufLe1StoreInfoCalc/7(LM_OTLCurLeLaObj2RcdFlg)
  LM_OTLCurObj2Dx/1 -> LM_OTL_BufLe1StoreInfoCalc/11(LM_OTLCurLeLaObj2Dx)
  LM_OTLBuf1ID/1 -> LM_OTL_BufLe1StoreInfoCalc/2(LM_OTLBuf1ID)

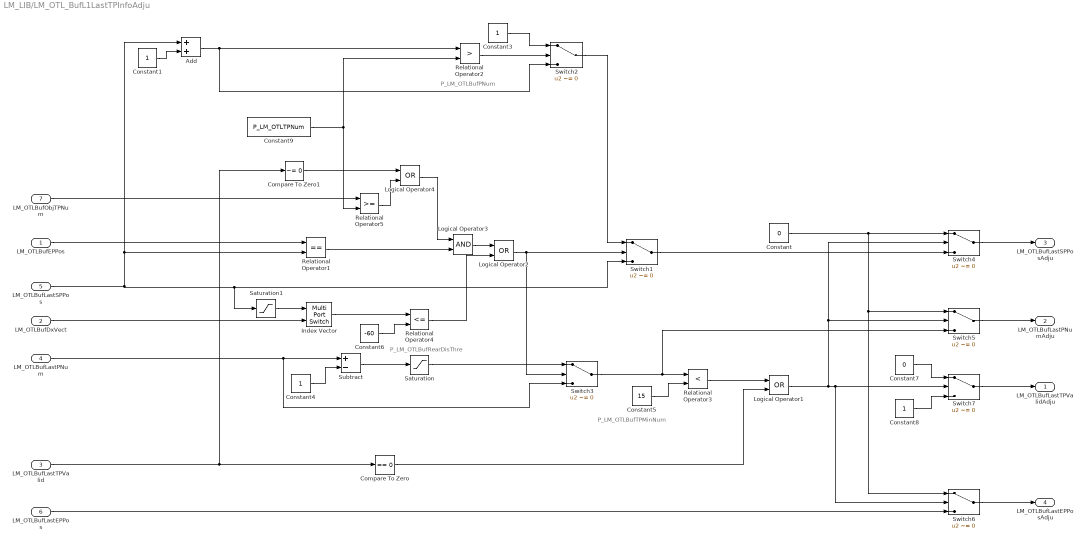
== system LM_LIB/LM_OTL_BufL1LastTPInfoAdju ==
  note: P_LM_OTLBufRearDisThre
  note: P_LM_OTLBufPNum
  note: P_LM_OTLBufTPMinNum
  LM_OTLBufEPPos : Inport
  LM_OTLBufDxVect : Inport  Port=2
  LM_OTLBufLastTPValid : Inport  Port=3
  LM_OTLBufLastPNum : Inport  Port=4
  LM_OTLBufLastSPPos : Inport  Port=5
  LM_OTLBufLastEPPos : Inport  Port=6
  LM_OTLBufObjTPNum : Inport  Port=7
  Add : Sum
  Compare To Zero : simulink/Logic and Bit Operations/Compare To Zero  relop===  OutDataTypeStr=boolean
  Compare To Zero1 : simulink/Logic and Bit Operations/Compare To Zero  relop=~=  OutDataTypeStr=boolean
  Constant : Constant  Value=0  OutDataTypeStr=uint8
  Constant{1,3..4,8} (4 alike) : Constant  OutDataTypeStr=uint8
  Constant5 : Constant  Value=15
  Constant6 : Constant  Value=-60  OutDataTypeStr=single
  Constant7 : Constant  Value=0  OutDataTypeStr=uint8
  Constant9 : Constant  Value=P_LM_OTLTPNum  OutDataTypeStr=uint8
  Index Vector : MultiPortSwitch  Inputs=1
  Logical Operator1 : Logic  Operator=OR  AllPortsSameDT=off  OutDataTypeStr=boolean
  Logical Operator2 : Logic  Operator=OR  AllPortsSameDT=off  OutDataTypeStr=boolean
  Logical Operator3 : Logic  AllPortsSameDT=off  OutDataTypeStr=boolean
  Logical Operator4 : Logic  Operator=OR  AllPortsSameDT=off  OutDataTypeStr=boolean
  Relational Operator1 : RelationalOperator  Operator===  OutDataTypeStr=boolean  RndMeth=Simplest
  Relational Operator2 : RelationalOperator  Operator=>  OutDataTypeStr=boolean  RndMeth=Simplest
  Relational Operator3 : RelationalOperator  Operator=<  OutDataTypeStr=boolean  RndMeth=Simplest
  Relational Operator4 : RelationalOperator  Operator=<=  OutDataTypeStr=boolean  RndMeth=Simplest
  Relational Operator5 : RelationalOperator  OutDataTypeStr=boolean  RndMeth=Simplest
  Saturation : Saturate  UpperLimit=80  LowerLimit=0
  Saturation1 : Saturate  UpperLimit=80  LowerLimit=1
  Subtract : Sum  Inputs=+-
  Switch{1..7} (7 alike) : Switch  Criteria=u2 ~= 0
  LM_OTLBufLastTPValidAdju : Outport  OutDataTypeStr=uint8  PortDimensions=1
  LM_OTLBufLastPNumAdju : Outport  Port=2  OutDataTypeStr=uint8  PortDimensions=1
  LM_OTLBufLastSPPosAdju : Outport  Port=3  OutDataTypeStr=uint8  PortDimensions=1
  LM_OTLBufLastEPPosAdju : Outport  Port=4  OutDataTypeStr=uint8  PortDimensions=1
  wires:
  Switch6/1 -> LM_OTLBufLastEPPosAdju/1
  LM_OTLBufLastEPPos/1 -> Switch6/3
  Switch4/1 -> LM_OTLBufLastSPPosAdju/1
  Switch5/1 -> LM_OTLBufLastPNumAdju/1
  Constant/1 -> Switch4/1, Switch5/1, Switch6/1
  Relational Operator4/1 -> Logical Operator2/2
  Relational Operator1/1 -> Logical Operator3/2
  Constant6/1 -> Relational Operator4/2
  Index Vector/1 -> Relational Operator4/1
  LM_OTLBufDxVect/1 -> Index Vector/2
  Logical Operator1/1 -> Switch4/2, Switch5/2, Switch6/2, Switch7/2
  LM_OTLBufLastTPValid/1 -> Compare To Zero1/1, Compare To Zero/1
  Relational Operator3/1 -> Logical Operator1/1
  Constant5/1 -> Relational Operator3/2
  Switch3/1 -> Relational Operator3/1, Switch5/3
  Saturation/1 -> Switch3/1
  Subtract/1 -> Saturation/1
  Constant4/1 -> Subtract/2
  LM_OTLBufLastPNum/1 -> Switch3/3, Subtract/1
  Switch2/1 -> Switch1/1
  Constant3/1 -> Switch2/1
  Switch1/1 -> Switch4/3
  Relational Operator2/1 -> Switch2/2
  Constant9/1 -> Relational Operator2/2, Relational Operator5/2
  Add/1 -> Relational Operator2/1, Switch2/3
  Constant1/1 -> Add/2
  Logical Operator2/1 -> Switch1/2, Switch3/2
  LM_OTLBufLastSPPos/1 -> Add/1, Relational Operator1/2, Saturation1/1, Switch1/3
  LM_OTLBufEPPos/1 -> Relational Operator1/1
  Saturation1/1 -> Index Vector/1
  Compare To Zero/1 -> Logical Operator1/2
  Switch7/1 -> LM_OTLBufLastTPValidAdju/1
  Constant7/1 -> Switch7/1
  Constant8/1 -> Switch7/3
  LM_OTLBufObjTPNum/1 -> Relational Operator5/1
  Relational Operator5/1 -> Logical Operator4/2
  Logical Operator3/1 -> Logical Operator2/1
  Compare To Zero1/1 -> Logical Operator4/1
  Logical Operator4/1 -> Logical Operator3/1

== system LM_LIB/LM_OTL_BufTPInfoEva ==
  LM_OTLBufDxVect : Inport
  LM_OTLBufDyVect : Inport  Port=2
  LM_OTLBufPNum : Inport  Port=3
  LM_OTLBufSPPos : Inport  Port=4
  LM_OTLBufEPPos : Inport  Port=5
  LM_OTLBufLastTPValid : Inport  Port=6
  LM_OTLBufLastPNum : Inport  Port=7
  LM_OTLBufLastSPPos : Inport  Port=8
  LM_OTLBufLastEPPos : Inport  Port=9
  LM_OTL_BufLe1TPInfoCalc : Subsystem
  LM_OTL_BufLe1TPPosInfo : Subsystem
  LM_OTL_BufLe1UsefulObjTPSelc : Subsystem
  LM_OTLBufValidTPNum : Outport
  LM_OTLBufValidSPPos : Outport  Port=2
  LM_OTLBufValidEPPos : Outport  Port=3
  wires:
  LM_OTL_BufLe1TPInfoCalc/2(LM_OTLBufL1ValidSPPos) -> LM_OTLBufValidSPPos/1  "LM_OTLBufValidSPPos"
  LM_OTL_BufLe1TPInfoCalc/1(LM_OTLBufL1ValidTPNum) -> LM_OTLBufValidTPNum/1  "LM_OTLBufValidTPNum"
  LM_OTL_BufLe1TPInfoCalc/3(LM_OTLBufL1ValidEPPos) -> LM_OTLBufValidEPPos/1  "LM_OTLBufValidEPPos"
  [LM_OTLBufL1SPPos] -> LM_OTL_BufLe1TPInfoCalc/3(LM_OTLBufL1SPPos)
  [LM_OTLBufL1PNum] -> LM_OTL_BufLe1TPInfoCalc/2(LM_OTLBufL1PNum)
  LM_OTL_BufLe1UsefulObjTPSelc/1(LM_OTLBufUsefulTPObjFlg) -> LM_OTL_BufLe1TPInfoCalc/1(LM_OTLBufUsefulTPObjFlg)
  LM_OTLBufLastPNum/1 -> LM_OTL_BufLe1TPInfoCalc/7(LM_OTLBufL1LastPNum), LM_OTL_BufLe1UsefulObjTPSelc/5(LM_OTLBufL1LastPNum)
  LM_OTL_BufLe1TPPosInfo/2(LM_OTLBufLe1LSOdxStart) -> LM_OTL_BufLe1UsefulObjTPSelc/2(LM_OTLBufLe1LSOdxStart)
  LM_OTL_BufLe1TPPosInfo/1(LM_OTLBufLe1CSOdxStart) -> LM_OTL_BufLe1UsefulObjTPSelc/1(LM_OTLBufLe1CSOdxStart)
  LM_OTLBufLastTPValid/1 -> LM_OTL_BufLe1UsefulObjTPSelc/4(LM_OTLBufL1LastTPValid), LM_OTL_BufLe1TPPosInfo/6(LM_OTLBufL1LastTPValid)
  LM_OTLBufLastEPPos/1 -> LM_OTL_BufLe1TPInfoCalc/6(LM_OTLBufL1LastEPPos), LM_OTL_BufLe1TPPosInfo/8(LM_OTLBufL1LastEPPos)
  LM_OTLBufLastSPPos/1 -> LM_OTL_BufLe1TPPosInfo/7(LM_OTLBufL1LastSPPos), LM_OTL_BufLe1TPInfoCalc/5(LM_OTLBufL1LastSPPos)
  LM_OTLBufEPPos/1 -> LM_OTL_BufLe1TPPosInfo/5(LM_OTLBufL1EPPos), LM_OTL_BufLe1TPInfoCalc/4(LM_OTLBufL1EPPos)
  LM_OTLBufSPPos/1 -> LM_OTL_BufLe1TPPosInfo/4(LM_OTLBufL1SPPos), [LM_OTLBufL1SPPos]
  LM_OTLBufPNum/1 -> LM_OTL_BufLe1UsefulObjTPSelc/3(LM_OTLBufL1PNum), LM_OTL_BufLe1TPPosInfo/3(LM_OTLBufL1PNum), [LM_OTLBufL1PNum]
  LM_OTLBufDyVect/1 -> LM_OTL_BufLe1TPPosInfo/2(LM_OTLBufL1DyVect)
  LM_OTLBufDxVect/1 -> LM_OTL_BufLe1TPPosInfo/1(LM_OTLBufL1DxVect)

== system LM_LIB/LM_EVOFusPath/LM_FusBLPathC0Calc ==
  LM_FusBLPathQuality : Inport
  LM_VSLPathP : Inport  Port=2
  LM_EMLPathP : Inport  Port=3
  LM_OTLPathP : Inport  Port=4
  LM_FusPathEMLK : Inport  Port=5
  LM_FusPathVSLK : Inport  Port=6
  LM_FusPathOTLK : Inport  Port=7
  Add : Sum
  Add5 : Sum
  Constant : Constant  Value=P_LM_FusParC0Index  OutDataTypeStr=uint8
  Constant1 : Constant  Value=0  OutDataTypeStr=single
  Constant2 : Constant  Value=0  OutDataTypeStr=single
  Index Vector : MultiPortSwitch  Inputs=1
  Index Vector1 : MultiPortSwitch  Inputs=1
  Index Vector8 : MultiPortSwitch  Inputs=1
  Product : Product
  Product1 : Product
  Product10 : Product
  Relational Operator : RelationalOperator  Operator===  OutDataTypeStr=boolean  RndMeth=Simplest
  Switch : Switch  Criteria=u2 ~= 0
  LM_FusBLPathC0 : Outport
  wires:
  Product1/1 -> Add/2
  Index Vector1/1 -> Product1/1
  Index Vector8/1 -> Product10/1
  LM_FusPathVSLK/1 -> Product/2
  LM_OTLPathP/1 -> Index Vector8/2
  LM_FusPathEMLK/1 -> Product1/2
  LM_EMLPathP/1 -> Index Vector1/2
  Product10/1 -> Add5/2
  LM_VSLPathP/1 -> Index Vector/2
  LM_FusPathOTLK/1 -> Product10/2
  Constant/1 -> Index Vector/1, Index Vector1/1, Index Vector8/1
  Index Vector/1 -> Product/1
  Add5/1 -> Switch/3  "LM_FusBLFntPath1C0"
  Product/1 -> Add/1
  Add/1 -> Add5/1  "LM_FusBLFntPath1C0"
  Constant1/1 -> Switch/1
  Constant2/1 -> Relational Operator/2
  LM_FusBLPathQuality/1 -> Relational Operator/1
  Switch/1 -> LM_FusBLPathC0/1  "LM_FusBLPathC0"
  Relational Operator/1 -> Switch/2

== system LM_LIB/LM_EVOFusPath/LM_FusBLPathC1Calc ==
  LM_FusBLPathQuality : Inport
  LM_VSLPathP : Inport  Port=2
  LM_EMLPathP : Inport  Port=3
  LM_OTLPathP : Inport  Port=4
  LM_FusPathEMLK : Inport  Port=5
  LM_FusPathVSLK : Inport  Port=6
  LM_FusPathOTLK : Inport  Port=7
  Add1 : Sum
  Add6 : Sum
  Constant1 : Constant  Value=P_LM_FusParC1Index  OutDataTypeStr=uint8
  Constant2 : Constant  Value=0  OutDataTypeStr=single
  Constant3 : Constant  Value=0  OutDataTypeStr=single
  Index Vector2 : MultiPortSwitch  Inputs=1
  Index Vector3 : MultiPortSwitch  Inputs=1
  Index Vector9 : MultiPortSwitch  Inputs=1
  Product11 : Product
  Product3 : Product
  Product4 : Product
  Relational Operator : RelationalOperator  Operator===  OutDataTypeStr=boolean  RndMeth=Simplest
  Switch : Switch  Criteria=u2 ~= 0
  LM_FusBLPathC1 : Outport
  wires:
  Index Vector2/1 -> Product3/1
  Index Vector3/1 -> Product4/1
  Product4/1 -> Add1/2
  Index Vector9/1 -> Product11/1
  LM_FusPathVSLK/1 -> Product3/2
  LM_OTLPathP/1 -> Index Vector9/2
  LM_FusPathEMLK/1 -> Product4/2
  LM_EMLPathP/1 -> Index Vector3/2
  Product11/1 -> Add6/2
  LM_VSLPathP/1 -> Index Vector2/2
  Add1/1 -> Add6/1  "LM_FusBLFntPath1C1"
  LM_FusPathOTLK/1 -> Product11/2
  Product3/1 -> Add1/1
  Constant1/1 -> Index Vector2/1, Index Vector3/1, Index Vector9/1
  Add6/1 -> Switch/3  "LM_FusBLFntPath1C0"
  Constant2/1 -> Switch/1
  Constant3/1 -> Relational Operator/2
  Relational Operator/1 -> Switch/2
  LM_FusBLPathQuality/1 -> Relational Operator/1
  Switch/1 -> LM_FusBLPathC1/1  "LM_FusBLPathC1"

== system LM_LIB/LM_EVOFusPath/LM_FusBLPathC2Calc ==
  LM_FusBLPathQuality : Inport
  LM_VSLPathP : Inport  Port=2
  LM_EMLPathP : Inport  Port=3
  LM_OTLPathP : Inport  Port=4
  LM_FusPathEMLK : Inport  Port=5
  LM_FusPathVSLK : Inport  Port=6
  LM_FusPathOTLK : Inport  Port=7
  Add2 : Sum
  Add7 : Sum
  Constant1 : Constant  Value=0  OutDataTypeStr=single
  Constant2 : Constant  Value=P_LM_FusParC2Index  OutDataTypeStr=uint8
  Constant3 : Constant  Value=0  OutDataTypeStr=single
  Index Vector10 : MultiPortSwitch  Inputs=1
  Index Vector4 : MultiPortSwitch  Inputs=1
  Index Vector5 : MultiPortSwitch  Inputs=1
  Product12 : Product
  Product2 : Product
  Product5 : Product
  Relational Operator : RelationalOperator  Operator===  OutDataTypeStr=boolean  RndMeth=Simplest
  Switch : Switch  Criteria=u2 ~= 0
  LM_FusBLPathC2 : Outport
  wires:
  Product2/1 -> Add2/1
  Index Vector5/1 -> Product5/1
  Index Vector10/1 -> Product12/1
  LM_FusPathVSLK/1 -> Product2/2
  LM_OTLPathP/1 -> Index Vector10/2
  LM_EMLPathP/1 -> Index Vector5/2
  LM_VSLPathP/1 -> Index Vector4/2
  LM_FusPathOTLK/1 -> Product12/2
  Add2/1 -> Add7/1  "LM_FusBLFntPath1C2"
  Product5/1 -> Add2/2
  Index Vector4/1 -> Product2/1
  LM_FusPathEMLK/1 -> Product5/2
  Product12/1 -> Add7/2
  Constant2/1 -> Index Vector4/1, Index Vector5/1, Index Vector10/1
  LM_FusBLPathQuality/1 -> Relational Operator/1
  Constant3/1 -> Relational Operator/2
  Relational Operator/1 -> Switch/2
  Constant1/1 -> Switch/1
  Switch/1 -> LM_FusBLPathC2/1  "LM_FusBLPathC2"
  Add7/1 -> Switch/3  "LM_FusBLFntPath1C2"

== system LM_LIB/LM_EVOFusPath/LM_FusBLPathC3Calc ==
  LM_FusBLPathQuality : Inport
  LM_VSLPathP : Inport  Port=2
  LM_EMLPathP : Inport  Port=3
  LM_OTLPathP : Inport  Port=4
  LM_FusPathEMLK : Inport  Port=5
  LM_FusPathVSLK : Inport  Port=6
  LM_FusPathOTLK : Inport  Port=7
  Add3 : Sum
  Add8 : Sum
  Constant1 : Constant  Value=0  OutDataTypeStr=single
  Constant2 : Constant  Value=0  OutDataTypeStr=single
  Constant3 : Constant  Value=P_LM_FusParC3Index  OutDataTypeStr=uint8
  Index Vector11 : MultiPortSwitch  Inputs=1
  Index Vector6 : MultiPortSwitch  Inputs=1
  Index Vector7 : MultiPortSwitch  Inputs=1
  Product13 : Product
  Product6 : Product
  Product7 : Product
  Relational Operator : RelationalOperator  Operator===  OutDataTypeStr=boolean  RndMeth=Simplest
  Switch : Switch  Criteria=u2 ~= 0
  LM_FusBLPathC3 : Outport
  wires:
  LM_FusPathOTLK/1 -> Product13/2
  LM_FusPathVSLK/1 -> Product6/2
  Product7/1 -> Add3/2
  LM_OTLPathP/1 -> Index Vector11/2
  LM_EMLPathP/1 -> Index Vector7/2
  LM_VSLPathP/1 -> Index Vector6/2
  LM_FusPathEMLK/1 -> Product7/2
  Constant3/1 -> Index Vector6/1, Index Vector7/1, Index Vector11/1
  Product13/1 -> Add8/2
  Index Vector11/1 -> Product13/1
  Index Vector7/1 -> Product7/1
  Add3/1 -> Add8/1  "LM_FusBLFntPath1C3"
  Index Vector6/1 -> Product6/1
  Product6/1 -> Add3/1
  Relational Operator/1 -> Switch/2
  Constant1/1 -> Switch/1
  Constant2/1 -> Relational Operator/2
  LM_FusBLPathQuality/1 -> Relational Operator/1
  Switch/1 -> LM_FusBLPathC3/1  "LM_FusBLPathC3"
  Add8/1 -> Switch/3

== system LM_LIB/LM_FusBLPathInfoFilt/LM_FusBLPathQuliatyFilt ==
  note: P_LM_FusBLParFiltP
  LM_FusBLPathQuality : Inport
  LM_FusBLPathQualityK1 : Inport  Port=2
  Add11 : Sum
  Compare To Zero : simulink/Logic and Bit Operations/Compare To Zero  relop=~=  OutDataTypeStr=boolean
  Compare To Zero1 : simulink/Logic and Bit Operations/Compare To Zero  relop===  OutDataTypeStr=boolean
  Compare To Zero2 : simulink/Logic and Bit Operations/Compare To Zero  relop===  OutDataTypeStr=boolean
  Constant9 : Constant  Value=P_LM_FusBLParFiltP  OutDataTypeStr=single
  Logical Operator : Logic  AllPortsSameDT=off  OutDataTypeStr=boolean
  MATLAB Function : MATLAB Function  TreatAsAtomicUnit=on
  Product16 : Product
  Subtract1 : Sum  Inputs=+-
  Switch1 : Switch  Criteria=u2 ~= 0
  Switch2 : Switch  Criteria=u2 ~= 0
  LM_FusBLPathQualityFilt : Outport
  wires:
  Switch2/1 -> MATLAB Function/1(u1)
  Compare To Zero2/1 -> Switch2/2
  Switch1/1 -> Switch2/3
  Logical Operator/1 -> Switch1/2
  Add11/1 -> Switch1/3  "LM_FusBLPathC1"
  LM_FusBLPathQuality/1 -> Compare To Zero2/1, Subtract1/1, Switch1/1, Compare To Zero/1, Switch2/1  "LM_FusBLFntPath1C0"
  LM_FusBLPathQualityK1/1 -> MATLAB Function/2(yk1), Add11/2, Subtract1/2, Compare To Zero1/1
  Product16/1 -> Add11/1
  Constant9/1 -> Product16/2
  Compare To Zero1/1 -> Logical Operator/2
  Subtract1/1 -> Product16/1
  MATLAB Function/1(y) -> LM_FusBLPathQualityFilt/1  "LM_FusBLPathQualityFilt"
  Compare To Zero/1 -> Logical Operator/1

== system LM_LIB/LM_FusBLPathInfoFilt/LM_Fus_BLFntPathC0Filt ==
  note: P_LM_FusBLParFiltP
  LM_FusBLPathC0 : Inport
  LM_FusBLPathQuality : Inport  Port=2
  LM_FusBLPathQualityK1 : Inport  Port=3
  LM_FusBLPathC0K1 : Inport  Port=4
  Add11 : Sum
  Compare To Zero : simulink/Logic and Bit Operations/Compare To Zero  relop=~=  OutDataTypeStr=boolean
  Compare To Zero1 : simulink/Logic and Bit Operations/Compare To Zero  relop===  OutDataTypeStr=boolean
  Constant9 : Constant  Value=P_LM_FusBLParFiltP  OutDataTypeStr=single
  Logical Operator : Logic  AllPortsSameDT=off  OutDataTypeStr=boolean
  MATLAB Function : MATLAB Function  TreatAsAtomicUnit=on
  Product16 : Product
  Subtract1 : Sum  Inputs=+-
  Switch1 : Switch  Criteria=u2 ~= 0
  LM_FusBLPathC0Filt : Outport
  wires:
  Compare To Zero1/1 -> Logical Operator/2
  LM_FusBLPathQualityK1/1 -> Compare To Zero1/1
  MATLAB Function/1(y) -> LM_FusBLPathC0Filt/1  "LM_FusBLPathC0Filt"
  Switch1/1 -> MATLAB Function/1(u1)
  Logical Operator/1 -> Switch1/2
  LM_FusBLPathC0K1/1 -> MATLAB Function/2(yk1), Add11/2, Subtract1/2
  Add11/1 -> Switch1/3  "LM_FusBLPathC1"
  LM_FusBLPathC0/1 -> Subtract1/1, Switch1/1  "LM_FusBLFntPath1C0"
  Constant9/1 -> Product16/2
  Subtract1/1 -> Product16/1
  Product16/1 -> Add11/1
  LM_FusBLPathQuality/1 -> Compare To Zero/1
  Compare To Zero/1 -> Logical Operator/1

== system LM_LIB/LM_FusBLPathInfoFilt/LM_Fus_BLPath3C3Filt ==
  note: P_LM_FusBLParFiltP
  LM_FusBLPathQualityK1 : Inport
  LM_FusBLPathQuality : Inport  Port=2
  LM_FusBLPathC3BefFilt : Inport  Port=3
  LM_FusBLPathC3K1 : Inport  Port=4
  Add11 : Sum
  Compare To Zero : simulink/Logic and Bit Operations/Compare To Zero  relop=~=  OutDataTypeStr=boolean
  Compare To Zero1 : simulink/Logic and Bit Operations/Compare To Zero  relop===  OutDataTypeStr=boolean
  Constant9 : Constant  Value=P_LM_FusBLParFiltP  OutDataTypeStr=single
  Logical Operator : Logic  AllPortsSameDT=off  OutDataTypeStr=boolean
  MATLAB Function : MATLAB Function  TreatAsAtomicUnit=on
  Product16 : Product
  Subtract1 : Sum  Inputs=+-
  Switch1 : Switch  Criteria=u2 ~= 0
  LM_FusBLPathC3Filt : Outport
  wires:
  Logical Operator/1 -> Switch1/2
  Add11/1 -> Switch1/3  "LM_FusBLPathC1"
  LM_FusBLPathC3BefFilt/1 -> Subtract1/1, Switch1/1  "LM_FusBLFntPath1C0"
  LM_FusBLPathC3K1/1 -> MATLAB Function/2(yk1), Add11/2, Subtract1/2
  Product16/1 -> Add11/1
  Constant9/1 -> Product16/2
  Compare To Zero1/1 -> Logical Operator/2
  Subtract1/1 -> Product16/1
  MATLAB Function/1(y) -> LM_FusBLPathC3Filt/1  "LM_FusBLPathC3Filt"
  Switch1/1 -> MATLAB Function/1(u1)
  LM_FusBLPathQuality/1 -> Compare To Zero/1
  Compare To Zero/1 -> Logical Operator/1
  LM_FusBLPathQualityK1/1 -> Compare To Zero1/1

== system LM_LIB/LM_FusBLPathInfoFilt/LM_Fus_BLPathC1Filt ==
  note: P_LM_FusBLParFiltP
  LM_FusBLPathQualityK1 : Inport
  LM_FusBLPathQuality : Inport  Port=2
  LM_FusBLPathC1BefFilt : Inport  Port=3
  LM_FusBLPathC1K1 : Inport  Port=4
  Add11 : Sum
  Compare To Zero : simulink/Logic and Bit Operations/Compare To Zero  relop=~=  OutDataTypeStr=boolean
  Compare To Zero1 : simulink/Logic and Bit Operations/Compare To Zero  relop===  OutDataTypeStr=boolean
  Constant9 : Constant  Value=P_LM_FusBLParFiltP  OutDataTypeStr=single
  Logical Operator : Logic  AllPortsSameDT=off  OutDataTypeStr=boolean
  MATLAB Function : MATLAB Function  TreatAsAtomicUnit=on
  Product16 : Product
  Subtract1 : Sum  Inputs=+-
  Switch1 : Switch  Criteria=u2 ~= 0
  LM_FusBLPathC1Filt : Outport
  wires:
  Logical Operator/1 -> Switch1/2
  Add11/1 -> Switch1/3  "LM_FusBLPathC1"
  LM_FusBLPathC1BefFilt/1 -> Subtract1/1, Switch1/1  "LM_FusBLFntPath1C0"
  LM_FusBLPathC1K1/1 -> MATLAB Function/2(yk1), Add11/2, Subtract1/2
  Product16/1 -> Add11/1
  Constant9/1 -> Product16/2
  Compare To Zero1/1 -> Logical Operator/2
  Subtract1/1 -> Product16/1
  MATLAB Function/1(y) -> LM_FusBLPathC1Filt/1  "LM_FusBLPathC1Filt"
  Switch1/1 -> MATLAB Function/1(u1)
  LM_FusBLPathQuality/1 -> Compare To Zero/1
  Compare To Zero/1 -> Logical Operator/1
  LM_FusBLPathQualityK1/1 -> Compare To Zero1/1

== system LM_LIB/LM_FusBLPathInfoFilt/LM_Fus_BLPathC2Filt ==
  note: P_LM_FusBLParFiltP
  LM_FusBLPathQualityK1 : Inport
  LM_FusBLPathQuality : Inport  Port=2
  LM_FusBLPathC2BefFilt : Inport  Port=3
  LM_FusBLPathC2K1 : Inport  Port=4
  Add11 : Sum
  Compare To Zero : simulink/Logic and Bit Operations/Compare To Zero  relop=~=  OutDataTypeStr=boolean
  Compare To Zero1 : simulink/Logic and Bit Operations/Compare To Zero  relop===  OutDataTypeStr=boolean
  Constant9 : Constant  Value=P_LM_FusBLParFiltP  OutDataTypeStr=single
  Logical Operator : Logic  AllPortsSameDT=off  OutDataTypeStr=boolean
  MATLAB Function : MATLAB Function  TreatAsAtomicUnit=on
  Product16 : Product
  Subtract1 : Sum  Inputs=+-
  Switch1 : Switch  Criteria=u2 ~= 0
  LM_FusBLPathC2Filt : Outport
  wires:
  LM_FusBLPathQualityK1/1 -> Compare To Zero1/1
  Compare To Zero/1 -> Logical Operator/1
  LM_FusBLPathQuality/1 -> Compare To Zero/1
  Switch1/1 -> MATLAB Function/1(u1)
  MATLAB Function/1(y) -> LM_FusBLPathC2Filt/1  "LM_FusBLPathC2Filt"
  Subtract1/1 -> Product16/1
  Compare To Zero1/1 -> Logical Operator/2
  Constant9/1 -> Product16/2
  Product16/1 -> Add11/1
  LM_FusBLPathC2K1/1 -> Subtract1/2, Add11/2, MATLAB Function/2(yk1)
  LM_FusBLPathC2BefFilt/1 -> Switch1/1, Subtract1/1  "LM_FusBLFntPath1C0"
  Add11/1 -> Switch1/3  "LM_FusBLPathC1"
  Logical Operator/1 -> Switch1/2
